simulink model "simulink_TA"  (R2023a)
settings: Solver=VariableStepAuto  StartTime=0.0  StopTime=1/24  RelTol=1e-3
values from neighbouring files (symbols this model uses):
  F = [F; Ca * (Aa^(i + 1))]    [get_F.m]
  H = P'*P+Rb    [get_H.m]
  P = [P; row]    [construct_P.m]
undefined symbols (not defined in the file or in its folder): A_cyc, A_kiln, B_cyc, B_kiln, C_cyc, C_kiln, C_kiln_mpc, control_horizon, F_cyc, F_kiln, H_cyc, H_kiln, P_cyc, P_kiln, prediction_horizon, u_fuel
libraries: simulink x3
settings Model: Creator=user  LastModifiedBy=user

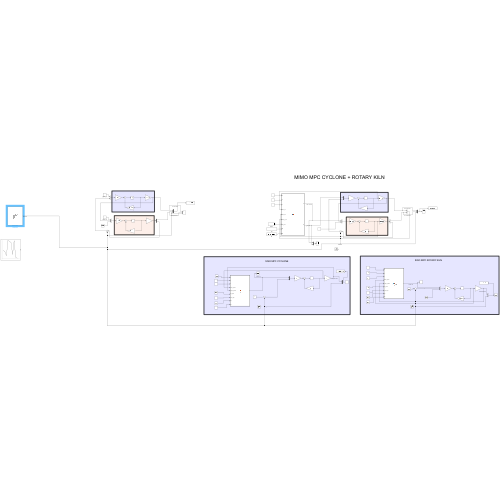
[thumbnail: Simulink's stored preview of the top-level diagram]
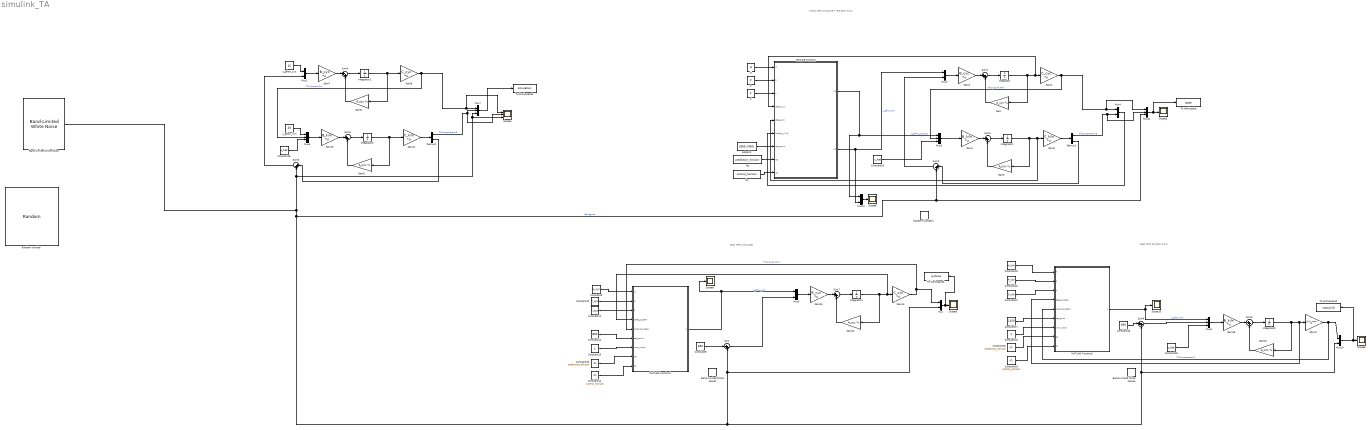
== system simulink_TA ==
  note: SISO MPC CYCLONE
  note: SISO MPC ROTARY KILN
  note: MIMO MPC CYCLONE + ROTARY KILN
  Band-Limited White Noise : simulink/Sources/Band-Limited White Noise  Cov=[400]  Ts=0.001  seed=[23341]
  Band-Limited White Noise1 : simulink/Sources/Band-Limited White Noise  Cov=[200]  Ts=0.001  seed=[23341]
  Band-Limited White Noise4 : simulink/Sources/Band-Limited White Noise  Cov=[200]  Ts=0.001  seed=[23341]
  Constant10 : Constant  Value=P_cyc
  Constant11 : Constant  Value=F_cyc
  Constant12 : Constant  Value=850
  Constant13 : Constant
  Constant14 : Constant  Value=control_horizon
  Constant15 : Constant  Value=prediction_horizon
  Constant16 : Constant  Value=850
  Constant17 : Constant  Value=1450
  Constant18 : Constant
  Constant19 : Constant  Value=control_horizon
  Constant20 : Constant  Value=prediction_horizon
  Constant21 : Constant  Value=F_kiln
  Constant22 : Constant  Value=P_kiln
  Constant23 : Constant  Value=H_kiln
  Constant24 : Constant  Value=u_fuel
  Constant25 : Constant  Value=u_fuel
  Constant26 : Constant  Value=u_fuel
  Constant8 : Constant  Value=850
  Constant9 : Constant  Value=H_cyc
  Demux1 : Demux  Outputs=2
  Demux2 : Demux  Outputs=2
  F : Constant  Value=F
  Gain : Gain  Gain=A_cyc  Multiplication=Matrix(K*u)
  Gain1 : Gain  Gain=B_cyc  Multiplication=Matrix(K*u)
  Gain10 : Gain  Gain=B_kiln  Multiplication=Matrix(K*u)
  Gain11 : Gain  Gain=C_kiln  Multiplication=Matrix(K*u)
  Gain12 : Gain  Gain=A_cyc  Multiplication=Matrix(K*u)
  Gain13 : Gain  Gain=B_cyc  Multiplication=Matrix(K*u)
  Gain14 : Gain  Gain=C_cyc  Multiplication=Matrix(K*u)
  Gain15 : Gain  Gain=A_kiln  Multiplication=Matrix(K*u)
  Gain16 : Gain  Gain=B_kiln  Multiplication=Matrix(K*u)
  Gain17 : Gain  Gain=C_kiln_mpc  Multiplication=Matrix(K*u)
  Gain2 : Gain  Gain=C_cyc  Multiplication=Matrix(K*u)
  Gain3 : Gain  Gain=A_kiln  Multiplication=Matrix(K*u)
  Gain4 : Gain  Gain=B_kiln  Multiplication=Matrix(K*u)
  Gain5 : Gain  Gain=C_kiln  Multiplication=Matrix(K*u)
  Gain6 : Gain  Gain=A_cyc  Multiplication=Matrix(K*u)
  Gain7 : Gain  Gain=B_cyc  Multiplication=Matrix(K*u)
  Gain8 : Gain  Gain=C_cyc  Multiplication=Matrix(K*u)
  Gain9 : Gain  Gain=A_kiln  Multiplication=Matrix(K*u)
  H : Constant  Value=H
  Integrator{,1..5} (6 alike) : Integrator
  MATLAB Function : MATLAB Function  TreatAsAtomicUnit=on
  MATLAB Function1 : MATLAB Function  TreatAsAtomicUnit=on
  MATLAB Function2 : MATLAB Function  TreatAsAtomicUnit=on
  Mux{,1..2,4..5,10,12} (7 alike) : Mux  Inputs=2
  Mux{3,6..7,9,11} (5 alike) : Mux  Inputs=3
  Nc : Constant  Value=control_horizon
  Np : Constant  Value=prediction_horizon
  P : Constant  Value=P
  Random Number : RandomNumber  Variance=10000  SampleTime=0.001
  Random Number1 : RandomNumber  Variance=500  SampleTime=0.001
  Scope{3,5..6,8..10} (6 alike) : Scope
  Scope4 : Scope  NumInputPorts=3
  Sum{,1..9} (10 alike) : Sum  Inputs=|++
  To Workspace : ToWorkspace  VariableName=state  SaveFormat=Timeseries  SampleTime=-1
  To Workspace1 : ToWorkspace  VariableName=cyclone  SaveFormat=Timeseries  SampleTime=-1
  To Workspace2 : ToWorkspace  VariableName=rotarykiln  SaveFormat=Timeseries  SampleTime=-1
  To Workspace3 : ToWorkspace  VariableName=simulation  SaveFormat=Timeseries  SampleTime=-1
  setpoint : Constant  Value=[850;1450]
  u_gflow_cyc : Constant  Value=10
  u_gflow_kiln : Constant  Value=40
  wires:
  Gain/1 -> Sum1/2
  Gain1/1 -> Sum1/1
  Mux2/1 -> Gain1/1
  MATLAB Function/2(u2) -> Mux12/2, Mux2/1  "u_gflow_kiln"
  Sum1/1 -> Integrator/1
  Gain2/1 -> Mux3/2, Mux11/1, Mux4/1  "Tf Cyclone Akhir"
  Sum2/1 -> Integrator1/1
  MATLAB Function/1(u1) -> Mux12/1, Mux3/1  "u_gflow_cyclone"
  Mux3/1 -> Gain4/1
  Integrator1/1 -> MATLAB Function/5(state_kiln), Gain5/1, Gain3/1
  Gain5/1 -> Demux1/1
  Gain4/1 -> Sum2/1
  Gain3/1 -> Sum2/2
  Demux1/2 -> Sum3/1
  H/1 -> MATLAB Function/1(H)
  F/1 -> MATLAB Function/3(F)
  setpoint/1 -> MATLAB Function/7(set_point)
  Np/1 -> MATLAB Function/8(Np)
  Integrator/1 -> MATLAB Function/4(state_cyc), Gain2/1, Gain/1
  P/1 -> MATLAB Function/2(P)
  Demux1/1 -> Mux11/2, Mux4/2  "Tf Compartment 3"
  Sum3/1 -> Mux2/2
  Gain9/1 -> Sum5/2
  Demux2/1 -> Scope4/2, Mux7/2  "Tf Compartment 3"
  Mux1/1 -> Gain7/1
  Gain11/1 -> Demux2/1
  Mux6/1 -> Gain10/1
  Sum6/1 -> Mux1/2
  Integrator3/1 -> Gain11/1, Gain9/1
  Gain7/1 -> Sum4/1
  Integrator2/1 -> Gain8/1, Gain6/1
  Gain10/1 -> Sum5/1
  Sum5/1 -> Integrator3/1
  Gain6/1 -> Sum4/2
  Sum4/1 -> Integrator2/1
  Demux2/2 -> Sum6/1
  Gain8/1 -> Mux6/2, Scope4/1, Mux7/1  "Tf Cyclone Akhir"
  u_gflow_kiln/1 -> Mux6/1
  u_gflow_cyc/1 -> Mux1/1
  Mux4/1 -> MATLAB Function/6(output_y1y2)
  Nc/1 -> MATLAB Function/9(Nc)
  Gain13/1 -> Sum7/1
  Mux5/1 -> Gain13/1
  Gain12/1 -> Sum7/2
  MATLAB Function1/1(u) -> Scope9/1, Mux5/1  "u_gflow_cyc"
  Sum7/1 -> Integrator4/1
  Integrator4/1 -> MATLAB Function1/4(state_system), Gain14/1, Gain12/1
  Constant8/1 -> Sum/1
  Gain14/1 -> Mux/1, MATLAB Function1/5(output_system)  "Tf Cyclone Akhir"
  Constant9/1 -> MATLAB Function1/1(H)
  Constant10/1 -> MATLAB Function1/2(P)
  Constant11/1 -> MATLAB Function1/3(F)
  Constant12/1 -> MATLAB Function1/6(set_point)
  Constant13/1 -> MATLAB Function1/7(num_input)
  Constant15/1 -> MATLAB Function1/8(Np)
  Constant14/1 -> MATLAB Function1/9(Nc)
  Sum8/1 -> Integrator5/1
  Gain16/1 -> Sum8/1
  Mux9/1 -> Gain16/1
  Gain15/1 -> Sum8/2
  MATLAB Function2/1(u) -> Mux9/1, Scope10/1  "u_gflow_kiln"
  Integrator5/1 -> MATLAB Function2/4(state_system), Gain17/1, Gain15/1
  Gain17/1 -> MATLAB Function2/5(output_system), Mux10/1  "Tf Compartment 3"
  Constant17/1 -> MATLAB Function2/6(set_point)
  Constant18/1 -> MATLAB Function2/7(num_input)
  Constant20/1 -> MATLAB Function2/8(Np)
  Constant19/1 -> MATLAB Function2/9(Nc)
  Constant21/1 -> MATLAB Function2/3(F)
  Constant22/1 -> MATLAB Function2/2(P)
  Constant23/1 -> MATLAB Function2/1(H)
  Constant24/1 -> Mux3/3
  Constant25/1 -> Mux9/3
  Constant26/1 -> Mux6/3
  Sum/1 -> Mux5/2
  Constant16/1 -> Sum9/1
  Sum9/1 -> Mux9/2
  Mux/1 -> To Workspace1/1, Scope5/1
  Mux10/1 -> To Workspace2/1, Scope6/1
  Mux11/1 -> To Workspace/1, Scope3/1
  Mux12/1 -> Scope8/1
  Band-Limited White Noise/1 -> Mux/2, Sum/2, Sum9/2, Mux10/2, Mux11/3, Sum3/2, Scope4/3, Mux7/3, Sum6/2  "Gangguan"
  Mux7/1 -> To Workspace3/1

== matlab function simulink_TA/MATLAB Function1 ==
  settings: updateMethod=DISCRETE  sampleTime=0.001
  data: H input; u output size=1; P input; F input; state_system input; output_system input; set_point input; num_input input; Np input; Nc input
function u  = custom_MPC(H, P, F, state_system, output_system, set_point, num_input, Np, Nc)

persistent states
if isempty(states)
   states=[zeros(size(state_system,1),1)];
else
   states=[states, state_system];
end

states = [states, state_system];
Rs = repmat(set_point, Np, 1);
xk = [states(:,end) - states(:,end-1);output_system];

f = -P'*(Rs - F*(xk));
options = optimoptions('quadprog','Algorithm','active-set');
lb = [0];
%[x, ~, Flag, Output] = quadprog(H, f,[],[],[],[],repmat(lb, Nc, 1),[],repmat(output_system, Nc, 1),options);
[x, ~, Flag, Output] = quadprog(H, f,[],[],[],[],[],[],repmat(output_system, Nc, 1),options);

u = x(1);
end

== matlab function simulink_TA/MATLAB Function ==
  settings: updateMethod=DISCRETE  sampleTime=0.001
  data: H input; u1 output size=1; P input; F input; state_cyc input; state_kiln input; output_y1y2 input; set_point input; Np input; u2 output size=1; Nc input
function [u1, u2] = custom_MPC(H, P, F, state_cyc, state_kiln, output_y1y2, set_point, Np, Nc)
current_state = [state_cyc ; state_kiln];

persistent states
if isempty(states)
   states=[zeros(16,1)];
else
   states=[states, current_state];
end

states = [states, current_state];
Rs = repmat(set_point, Np, 1);
xk = [states(:,end) - states(:,end-1);output_y1y2];

f = -P'*(Rs - F*(xk));
options = optimoptions('quadprog','Algorithm','active-set');


% without constrain
[x, ~, Flag, Output] = quadprog(H, f,[],[],[],[],[],[],repmat(output_y1y2, Nc, 1),options);

% adding constrain

% lb = [0; 0]; % minimum values for input result
% % Define the output constraints
% y_min = [0; 0];  % Minimum values for the outputs
% y_max = [900; 2000];  % Maximum values for the outputs
% b_output = [y_max; -y_min];
% C_c = [0, 0, 0, 1, 0, 0, 0, 0, 0, 0, 0, 0, 0, 0, 0, 0; 
%        0, 0, 0, 0, 0, 0, 0, 0, 0, 0, 1, 0, 0, 0, 0, 0];
% A_output = eye(8);
%[x, ~, Flag, Output] = quadprog(H, f,repmat(A_output, Nc, 1),b_output,[],[],repmat(lb, Nc, 1),[],repmat(output_y1y2, Nc, 1),options);

u1 = x(1);
u2 = x(2);
end

== matlab function simulink_TA/MATLAB Function2 ==
  settings: updateMethod=DISCRETE  sampleTime=0.001
  data: H input; u output size=1; P input; F input; state_system input; output_system input; set_point input; num_input input; Np input; Nc input
function u  = custom_MPC(H, P, F, state_system, output_system, set_point, num_input, Np, Nc)

persistent states
if isempty(states)
   states=[zeros(size(state_system,1),1)];
else
   states=[states, state_system];
end

states = [states, state_system];
Rs = repmat(set_point, Np, 1);
xk = [states(:,end) - states(:,end-1);output_system];

f = -P'*(Rs - F*(xk));
options = optimoptions('quadprog','Algorithm','active-set');
lb = [0];
%[x, ~, Flag, Output] = quadprog(H, f,[],[],[],[],repmat(lb, Nc, 1),[],repmat(output_system, Nc, 1),options);
[x, ~, Flag, Output] = quadprog(H, f,[],[],[],[],[],[],repmat(output_system, Nc, 1),options);

u = x(1);
end
